simulink model "sim_switch_vol_hover"  (R2020b)
settings: Solver=VariableStepAuto  StartTime=0.0  StopTime=T  MaxStep=MaxStep  RelTol=RelTol
values from neighbouring files (symbols this model uses):
  a = 400    [switch_vol_hovering.m]
  b = 500    [switch_vol_hovering.m]
  drone = generateDarko()    [switch_vol_hovering.m]
  J = 200    [switch_vol_hovering.m]
  K_complet = [K(:,1:6), [0;0;0;0], K(:,7:12)]    [switch_vol_hovering.m]
  K_lin_control = [zeros(4,2), K_lin(:,1:4), zeros(4,1), K_lin(:,5:10)]    [switch_vol_hovering.m]
  position_cible = [50; 0; 0]    [switch_vol_hovering.m]
  rule = 1    [switch_vol_hovering.m]
  S_complet = [S(1:6,1:6), zeros(6,1), S(1:6,7:12); zeros(1,13); S(7:12,1:6), zeros(6,1), S(7:12,7:12)]    [switch_vol_hovering.m]
  T = 80    [switch_vol_hovering.m]
  u_eq_hover = drone.G*drone.MASS/(2*drone.Fb(1,1)) * [1;1;0;0]    [switch_vol_hovering.m]
  u_eq_vol = [trim(1);trim(1);trim(2);trim(2)]    [switch_vol_hovering.m]
  x0 = [p_initial; v_initial; q_initial; omega_initial; s]    [switch_vol_hovering.m]
  x_eq_hover = [[0; 0; 0]; [0; 0; 0]; [1/sqrt(2); 0; -1/sqrt(2);0]; [0; 0; 0]]    [switch_vol_hovering.m]
  x_eq_vol = [p_initial; v_initial; q_initial; omega_initial]    [switch_vol_hovering.m]
libraries: simulink x3, simulink_extras x3, aerolibanim x1, sharedtransform x1
settings Model: Creator=florian  LastModifiedBy=florian

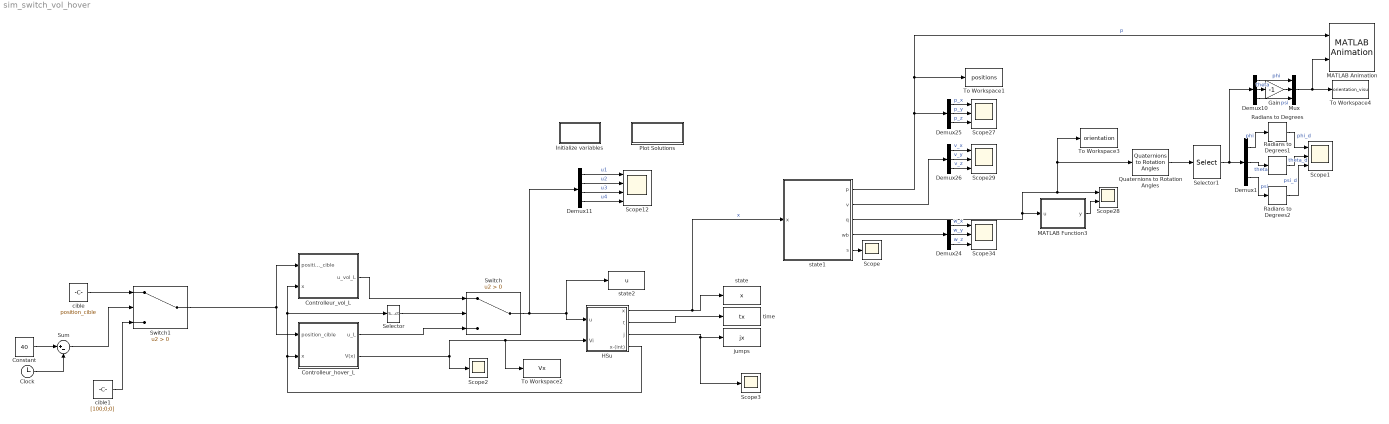
== system sim_switch_vol_hover ==
  Clock : Clock
  Constant : Constant  Value=40
  Controlleur_hover_L : Subsystem
  Controlleur_vol_L : Subsystem
  Demux{1,10,24..26} (5 alike) : Demux  Outputs=3
  Demux11 : Demux
  Gain : Gain  Gain=-1
  HSu : Subsystem  LoadFcn=set_param(gcb,'LinkStatus','none')
      settings: CopyFcn=|
      | set_param(gcb,'LinkStatus','none'),
      | set_param(gcs, 'MaxStep', 'MaxStep', 'RelTol', 'RelTol','Stop time', 'T')
      mask Display:
      | image(imread('Hcal.jpg'))
      | %plot([5 20 20 5 5],[5 5 20 20 5])
      | %text(8,13,'HyEq_mdl')
      | port_label('output', 1, 'x')
      | port_label('output', 2, 't')
      | port_label('output', 3, 'j')
      | port_label('output', 4, 'x-(int)')
      | port_label('input', 1, 'u')
      | port_label('input', 2, 'V(x)')
  Initialize variables : Subsystem  Priority=-10
      settings: OpenFcn=initialization_di
      mask Display: disp('Double Click\n to Initialize')
  MATLAB Animation : aerolibanim/MATLAB Animation  Tag=Matlab Animation 6 DOF  Vehicles=1  Geometries='astredwedge.mat'  BoundingBoxCoordinates=[-50,50,-50,50,-50,50]  CameraOffset=[-150,-50,0]  CameraViewAngle=3  SampleTime=0.2  FigurePosition=[962,411,639,384]
      settings: SourceProductBaseCode=AE
  MATLAB Function3 : MATLAB Function  TreatAsAtomicUnit=on
  Mux : Mux  Inputs=3
  Plot Solutions : Subsystem
      settings: OpenFcn=postprocessing_di
      mask Display: disp('Double Click to\n Plot Solutions')
  Quaternions to Rotation Angles : sharedtransform/Quaternions to Rotation Angles  rotationOrder=ZXY  aMode=aMode
      settings: SourceProductBaseCode=AE,PW,MT,UV,VE,VP
  Radians to Degrees : simulink_extras/Transformations/Radians to Degrees
  Radians to Degrees1 : simulink_extras/Transformations/Radians to Degrees
  Radians to Degrees2 : simulink_extras/Transformations/Radians to Degrees
  Scope : Scope
  Scope{1,27,29,34} (4 alike) : Scope  NumInputPorts=3
  Scope12 : Scope  NumInputPorts=4
  Scope2 : Scope
  Scope28 : Scope  NumInputPorts=2
  Scope3 : Scope
  Selector : Selector  InputPortWidth=14  IndexOptions=Index vector (dialog)  Indices=[14]  OutputSizes=1
  Selector1 : Selector  InputPortWidth=3  IndexOptions=Index vector (dialog)  Indices=[2 3 1]  OutputSizes=1
  Sum : Sum  Inputs=|+-
  Switch : Switch  Criteria=u2 > Threshold
  Switch1 : Switch  Criteria=u2 > Threshold
  To Workspace1 : ToWorkspace  VariableName=positions  SampleTime=-1
  To Workspace2 : ToWorkspace  VariableName=Vx  SampleTime=-1
  To Workspace3 : ToWorkspace  VariableName=orientation  SampleTime=-1
  To Workspace4 : ToWorkspace  VariableName=orientation_visu  SampleTime=-1
  cible : Constant  Value=position_cible
  cible1 : Constant  Value=[100;0;0]
  jumps : ToWorkspace  VariableName=jx  SampleTime=-1
  state : ToWorkspace  VariableName=x  SampleTime=-1
  state1 : MATLAB Function  TreatAsAtomicUnit=on
  state2 : ToWorkspace  VariableName=u  SampleTime=-1
  time : ToWorkspace  VariableName=tx  SampleTime=-1
  wires:
  Switch/1 -> HSu/1(u), state2/1, Demux11/1
  HSu/1(x) -> state1/1(x), state/1  "x"
  HSu/2(t) -> time/1
  HSu/3(j) -> jumps/1, Scope3/1
  Demux11/2 -> Scope12/2  "u2"
  Controlleur_vol_L/1(u_vol_L) -> Switch/1
  Controlleur_hover_L/1(u_L) -> Switch/3
  Demux11/1 -> Scope12/1  "u1"
  Demux11/4 -> Scope12/4  "u4"
  Switch1/1 -> Controlleur_vol_L/1(position_cible), Controlleur_hover_L/1(position_cible)
  Demux11/3 -> Scope12/3  "u3"
  Selector/1 -> Switch/2
  HSu/4(x-(int)) -> Controlleur_vol_L/2(x), Selector/1, Controlleur_hover_L/2(x)
  Demux1/2 -> Radians to Degrees1/1  "theta"
  Quaternions to Rotation Angles/1 -> Selector1/1
  Demux1/3 -> Radians to Degrees2/1  "psi"
  Demux24/2 -> Scope34/2  "w_y"
  Demux26/3 -> Scope29/3  "v_z"
  Demux25/3 -> Scope27/3  "p_z"
  Demux1/1 -> Radians to Degrees/1  "phi"
  Demux25/1 -> Scope27/1  "p_x"
  state1/3(q) -> Scope28/1, To Workspace3/1, Quaternions to Rotation Angles/1, MATLAB Function3/1(u)
  Radians to Degrees/1 -> Scope1/1  "phi_d"
  Radians to Degrees1/1 -> Scope1/2  "theta_d"
  Radians to Degrees2/1 -> Scope1/3  "psi_d"
  MATLAB Function3/1(y) -> Scope28/2
  state1/2(v) -> Demux26/1
  Demux26/2 -> Scope29/2  "v_y"
  Demux24/3 -> Scope34/3  "w_z"
  state1/4(wb) -> Demux24/1
  Demux24/1 -> Scope34/1  "w_x"
  Demux26/1 -> Scope29/1  "v_x"
  Demux25/2 -> Scope27/2  "p_y"
  state1/5(s) -> Scope/1
  cible/1 -> Switch1/1
  Constant/1 -> Sum/1
  Clock/1 -> Sum/2
  Sum/1 -> Switch1/2
  cible1/1 -> Switch1/3
  Controlleur_hover_L/2(V(x)) -> Scope2/1, To Workspace2/1, HSu/2(Vi)
  Gain/1 -> Mux/2
  Demux10/1 -> Mux/1  "phi"
  Demux10/2 -> Gain/1  "theta"
  Demux10/3 -> Mux/3  "psi"
  state1/1(p) -> MATLAB Animation/1, To Workspace1/1, Demux25/1  "p"
  Selector1/1 -> Demux10/1, Demux1/1
  Mux/1 -> To Workspace4/1, MATLAB Animation/2

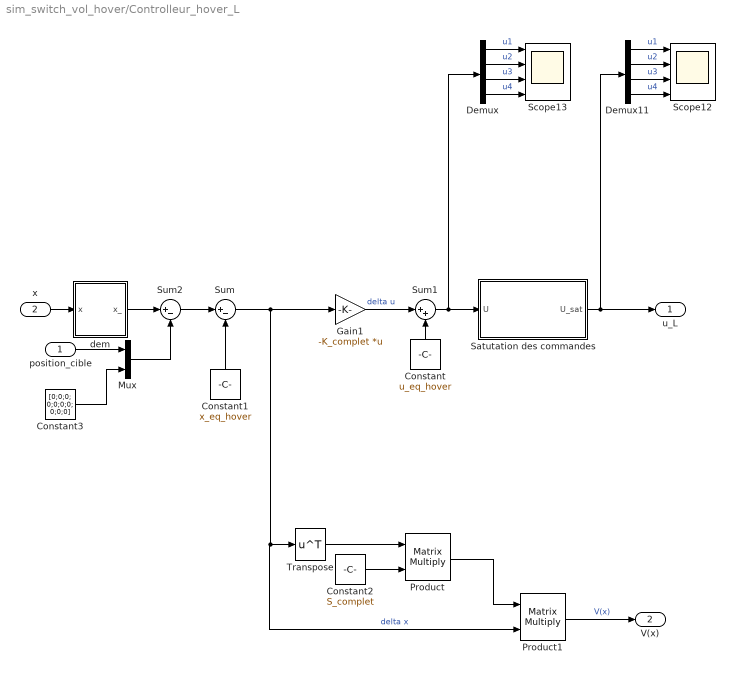
== system sim_switch_vol_hover/Controlleur_hover_L ==
  position_cible : Inport
  x : Inport  Port=2
  Constant : Constant  Value=u_eq_hover
  Constant1 : Constant  Value=x_eq_hover
  Constant2 : Constant  Value=S_complet
  Constant3 : Constant  Value=[0;0;0; 0;0;0;0; 0;0;0]
  Demux : Demux
  Demux11 : Demux
  Gain1 : Gain  Gain=-K_complet  Multiplication=Matrix(K*u) (u vector)
  Mux : Mux  Inputs=2
  Product : Product  Multiplication=Matrix(*)
  Product1 : Product  Multiplication=Matrix(*)
  Satutation des commandes : Subsystem
  Scope12 : Scope  NumInputPorts=4
  Scope13 : Scope  NumInputPorts=4
  Sum : Sum  Inputs=|+-
  Sum1 : Sum  Inputs=|++
  Sum2 : Sum  Inputs=|+-
  Transpose : Math  Operator=transpose  SaturateOnIntegerOverflow=on
  dem : MATLAB Function  TreatAsAtomicUnit=on
  u_L : Outport
  V(x) : Outport  Port=2
  wires:
  Demux/1 -> Scope13/1  "u1"
  Demux/3 -> Scope13/3  "u3"
  Gain1/1 -> Sum1/1  "delta u"
  Sum1/1 -> Satutation des commandes/1(U), Demux/1
  Sum/1 -> Gain1/1, Product1/2, Transpose/1  "delta x"
  Demux11/3 -> Scope12/3  "u3"
  Satutation des commandes/1(U_sat) -> u_L/1, Demux11/1
  Demux11/2 -> Scope12/2  "u2"
  Product1/1 -> V(x)/1  "V(x)"
  Demux/4 -> Scope13/4  "u4"
  Constant1/1 -> Sum/2
  Transpose/1 -> Product/1
  Product/1 -> Product1/1
  Constant/1 -> Sum1/2
  Demux11/4 -> Scope12/4  "u4"
  Demux/2 -> Scope13/2  "u2"
  Constant2/1 -> Product/2
  Sum2/1 -> Sum/1
  Demux11/1 -> Scope12/1  "u1"
  Mux/1 -> Sum2/2
  position_cible/1 -> Mux/1
  Constant3/1 -> Mux/2
  x/1 -> dem/1(x)
  dem/1(x_) -> Sum2/1

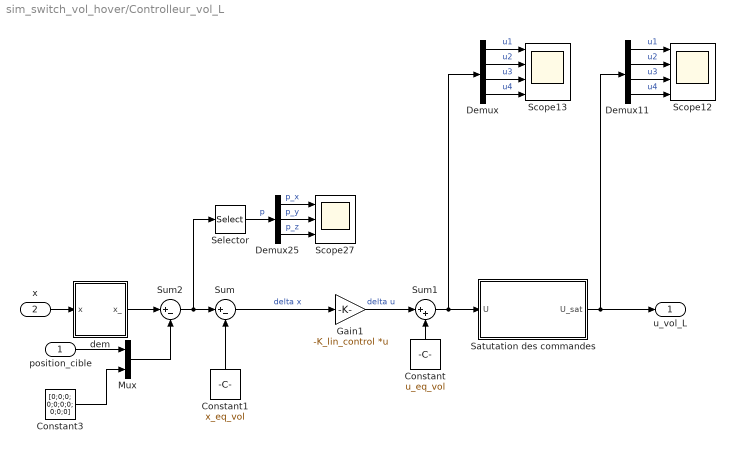
== system sim_switch_vol_hover/Controlleur_vol_L ==
  position_cible : Inport
  x : Inport  Port=2
  Constant : Constant  Value=u_eq_vol
  Constant1 : Constant  Value=x_eq_vol
  Constant3 : Constant  Value=[0;0;0; 0;0;0;0; 0;0;0]
  Demux : Demux
  Demux11 : Demux
  Demux25 : Demux  Outputs=3
  Gain1 : Gain  Gain=-K_lin_control  Multiplication=Matrix(K*u) (u vector)
  Mux : Mux  Inputs=2
  Satutation des commandes : Subsystem
  Scope12 : Scope  NumInputPorts=4
  Scope13 : Scope  NumInputPorts=4
  Scope27 : Scope  NumInputPorts=3
  Selector : Selector  InputPortWidth=13  IndexOptions=Index vector (dialog)  Indices=[1 2 3]  OutputSizes=1
  Sum : Sum  Inputs=|+-
  Sum1 : Sum  Inputs=|++
  Sum2 : Sum  Inputs=|+-
  dem : MATLAB Function  TreatAsAtomicUnit=on
  u_vol_L : Outport
  wires:
  Demux/1 -> Scope13/1  "u1"
  Demux/3 -> Scope13/3  "u3"
  Gain1/1 -> Sum1/1  "delta u"
  Sum1/1 -> Satutation des commandes/1(U), Demux/1
  Sum/1 -> Gain1/1  "delta x"
  Demux11/3 -> Scope12/3  "u3"
  Satutation des commandes/1(U_sat) -> u_vol_L/1, Demux11/1
  Demux11/2 -> Scope12/2  "u2"
  Demux/4 -> Scope13/4  "u4"
  Constant1/1 -> Sum/2
  Constant/1 -> Sum1/2
  Demux11/4 -> Scope12/4  "u4"
  Demux/2 -> Scope13/2  "u2"
  Sum2/1 -> Selector/1, Sum/1
  Demux11/1 -> Scope12/1  "u1"
  Mux/1 -> Sum2/2
  position_cible/1 -> Mux/1
  Constant3/1 -> Mux/2
  x/1 -> dem/1(x)
  dem/1(x_) -> Sum2/1
  Demux25/3 -> Scope27/3  "p_z"
  Demux25/1 -> Scope27/1  "p_x"
  Selector/1 -> Demux25/1  "p"
  Demux25/2 -> Scope27/2  "p_y"

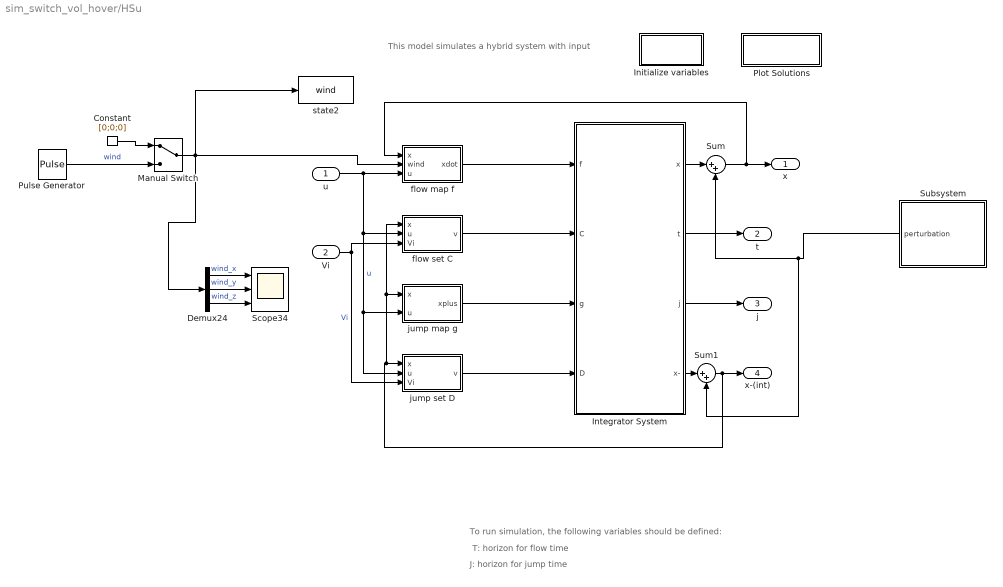
== system sim_switch_vol_hover/HSu ==
  note: J: horizon for jump time
  note: T: horizon for flow time
  note: To run simulation, the following variables should be defined:
  note: This model simulates a hybrid system with input
  u : Inport
  Vi : Inport  Port=2
  Constant : Constant  Value=[0;0;0]
  Demux24 : Demux  Outputs=3
  Initialize variables : Subsystem  Priority=-10
      settings: OpenFcn=|
      | try
      |      clearvars -except inifile pathfile_in pathfile_pos posfile
      |      cd(pathfile_in);
      |      eval(inifile);
      | catch
      |      [inifile,pathfile_in] = getInitializationfile;
      |      cd(pathfile_in);
      |      inifile = strrep(inifile,'.m','');
      |      eval(inifile);
      | end
      mask Display: disp('Double Click\n to Initialize')
  Integrator System : Subsystem  Priority=2  mask(Hybrid Integrator){T=T, J=J, x0=x0}
      mask prompts: T "Flow Horizon"; J "Jump Horizon"; x0 "Initial Condition"
      mask help:
      | This block integrates the state of the hybrid system defined by the flow map f (first input), the flow set C (second input), the jump map g (third input) and the jump set D (fourth input).
      | Starting from the initial condition x0 (last mask parameter), the system's state x evolves continuously within the set C, according to f(x,u), but is also subject to jumps within D, according to g(x,u).
      | The block also stops the simulation when the time t is greater than the flow horizon T (first mask parameter), or when the number of jumps j is greater than the jump horizon J (second mask parameter).
      | The outputs of the blocks are respectively x(t), t, j, x(t-).
      mask Help:
      | This block integrates the state of the hybrid system defined by the flow map f (first input), the flow set C (second input), the jump map g (third input) and the jump set D (fourth input).
      | <br>
      | Starting from the initial condition x0 (last mask parameter), the system's state x evolves continuously within the set C, according to f(x,u), but is also subject to jumps within D, according to g(x,u).
      | <br>
      | The block also stops the simulation when the time t is greater than the flow horizon T (first mask parameter), or when the number of jumps j is greater than the jump horizon J (second mask parameter).
      | <br>
      | The outputs of the blocks are respectively x(t), t, j, x(t-).
      | <br>
      | You can right click on the block and "Look under mask" to see what's inside the block.
      | Finally, refer to the manual (HybridSimulator_vXX.pdf) for more detailed information on how this hybrid simulator works.
  Manual Switch : ManualSwitch
  Plot Solutions : Subsystem
      settings: OpenFcn=|
      | try
      |      cd(pathfile_pos);
      |      eval(posfile);
      | catch
      |      [posfile,pathfile_pos] = getInitializationfile;
      |      cd(pathfile_pos);
      |      posfile = strrep(posfile,'.m','');
      |      eval(posfile);
      | end
      mask Display: disp('Double Click to\n Plot Solutions')
  Pulse Generator : DiscretePulseGenerator  PulseType=Time based  Amplitude=1.9  Period=10  PulseWidth=30  PhaseDelay=5
  Scope34 : Scope  NumInputPorts=3
  Subsystem : Subsystem
  Sum : Sum  Inputs=|++
  Sum1 : Sum  Inputs=|++
  flow map f : MATLAB Function  TreatAsAtomicUnit=on
  flow set C : MATLAB Function  TreatAsAtomicUnit=on
  jump map g : MATLAB Function  Priority=2  TreatAsAtomicUnit=on
  jump set D : MATLAB Function  TreatAsAtomicUnit=on
  state2 : ToWorkspace  VariableName=wind  SampleTime=-1
  x : Outport
  t : Outport  Port=2
  j : Outport  Port=3
  x-(int) : Outport  Port=4
  wires:
  jump map g/1(xplus) -> Integrator System/3(g)
  jump set D/1(v) -> Integrator System/4(D)
  u/1 -> jump set D/2(u), jump map g/2(u), flow set C/2(u), flow map f/3(u)  "u"
  Integrator System/3(j) -> j/1
  Integrator System/2(t) -> t/1
  flow set C/1(v) -> Integrator System/2(C)
  flow map f/1(xdot) -> Integrator System/1(f)
  Vi/1 -> jump set D/3(Vi), flow set C/3(Vi)  "Vi"
  Constant/1 -> Manual Switch/1
  Manual Switch/1 -> Demux24/1, state2/1, flow map f/2(wind)
  Demux24/1 -> Scope34/1  "wind_x"
  Demux24/2 -> Scope34/2  "wind_y"
  Demux24/3 -> Scope34/3  "wind_z"
  Pulse Generator/1 -> Manual Switch/2  "wind"
  Sum1/1 -> flow set C/1(x), jump map g/1(x), jump set D/1(x), x-(int)/1
  Subsystem/1(perturbation) -> Sum/2, Sum1/2
  Integrator System/1(x) -> Sum/1
  Sum/1 -> flow map f/1(x), x/1
  Integrator System/4(x-) -> Sum1/1

== system sim_switch_vol_hover/Initialize variables ==

== system sim_switch_vol_hover/Plot Solutions ==

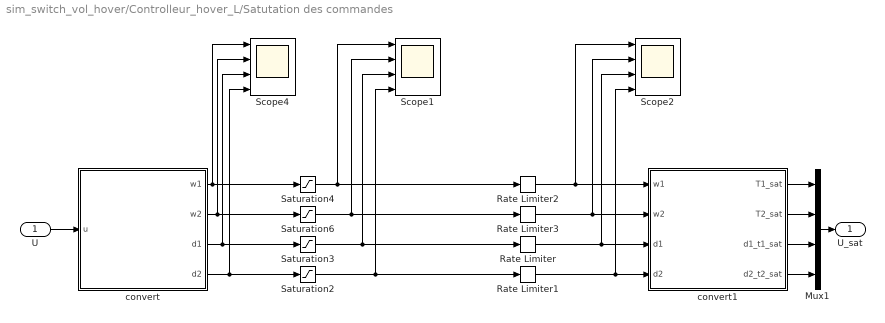
== system sim_switch_vol_hover/Controlleur_hover_L/Satutation des commandes ==
  U : Inport
  Mux1 : Mux
  Rate Limiter : RateLimiter  RisingSlewLimit=drone.ELEVON_RATE_CHANGE  FallingSlewLimit=-drone.ELEVON_RATE_CHANGE  SampleTimeMode=inherited
  Rate Limiter1 : RateLimiter  RisingSlewLimit=drone.ELEVON_RATE_CHANGE  FallingSlewLimit=-drone.ELEVON_RATE_CHANGE  SampleTimeMode=inherited
  Rate Limiter2 : RateLimiter  RisingSlewLimit=drone.MOTOR_RATE_CHANGE  FallingSlewLimit=-drone.MOTOR_RATE_CHANGE  SampleTimeMode=inherited
  Rate Limiter3 : RateLimiter  RisingSlewLimit=drone.MOTOR_RATE_CHANGE  FallingSlewLimit=-drone.MOTOR_RATE_CHANGE  SampleTimeMode=inherited
  Saturation2 : Saturate  UpperLimit=30*(pi/180)  LowerLimit=-30*(pi/180)
  Saturation3 : Saturate  UpperLimit=30*(pi/180)  LowerLimit=-30*(pi/180)
  Saturation4 : Saturate  UpperLimit=1000  LowerLimit=200
  Saturation6 : Saturate  UpperLimit=1000  LowerLimit=200
  Scope1 : Scope  NumInputPorts=4
  Scope2 : Scope  NumInputPorts=4
  Scope4 : Scope  NumInputPorts=4
  convert : MATLAB Function  TreatAsAtomicUnit=on
  convert1 : MATLAB Function  TreatAsAtomicUnit=on
  U_sat : Outport
  wires:
  convert/1(w1) -> Saturation4/1, Scope4/1
  Saturation3/1 -> Rate Limiter/1, Scope1/3
  convert/2(w2) -> Scope4/2, Saturation6/1
  convert/3(d1) -> Scope4/3, Saturation3/1
  convert/4(d2) -> Saturation2/1, Scope4/4
  convert1/1(T1_sat) -> Mux1/1
  convert1/4(d2_t2_sat) -> Mux1/4
  Mux1/1 -> U_sat/1
  convert1/2(T2_sat) -> Mux1/2
  convert1/3(d1_t1_sat) -> Mux1/3
  Saturation2/1 -> Rate Limiter1/1, Scope1/4
  Rate Limiter/1 -> Scope2/3, convert1/3(d1)
  Saturation6/1 -> Rate Limiter3/1, Scope1/2
  Saturation4/1 -> Rate Limiter2/1, Scope1/1
  Rate Limiter1/1 -> Scope2/4, convert1/4(d2)
  Rate Limiter2/1 -> Scope2/1, convert1/1(w1)
  Rate Limiter3/1 -> Scope2/2, convert1/2(w2)
  U/1 -> convert/1(u)

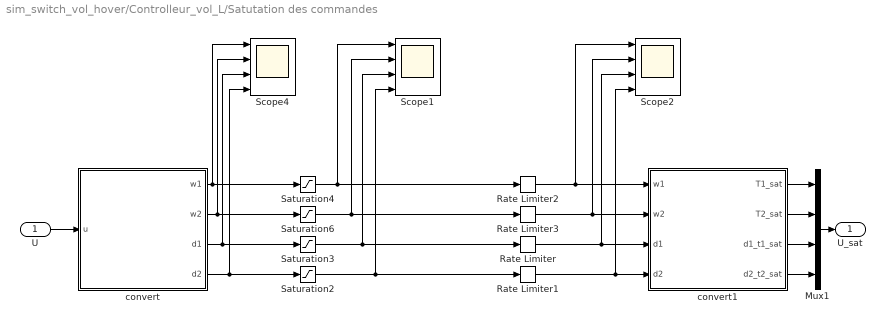
== system sim_switch_vol_hover/Controlleur_vol_L/Satutation des commandes ==
  U : Inport
  Mux1 : Mux
  Rate Limiter : RateLimiter  RisingSlewLimit=drone.ELEVON_RATE_CHANGE  FallingSlewLimit=-drone.ELEVON_RATE_CHANGE  SampleTimeMode=inherited
  Rate Limiter1 : RateLimiter  RisingSlewLimit=drone.ELEVON_RATE_CHANGE  FallingSlewLimit=-drone.ELEVON_RATE_CHANGE  SampleTimeMode=inherited
  Rate Limiter2 : RateLimiter  RisingSlewLimit=drone.MOTOR_RATE_CHANGE  FallingSlewLimit=-drone.MOTOR_RATE_CHANGE  SampleTimeMode=inherited
  Rate Limiter3 : RateLimiter  RisingSlewLimit=drone.MOTOR_RATE_CHANGE  FallingSlewLimit=-drone.MOTOR_RATE_CHANGE  SampleTimeMode=inherited
  Saturation2 : Saturate  UpperLimit=30*(pi/180)  LowerLimit=-30*(pi/180)
  Saturation3 : Saturate  UpperLimit=30*(pi/180)  LowerLimit=-30*(pi/180)
  Saturation4 : Saturate  UpperLimit=1000  LowerLimit=200
  Saturation6 : Saturate  UpperLimit=1000  LowerLimit=200
  Scope1 : Scope  NumInputPorts=4
  Scope2 : Scope  NumInputPorts=4
  Scope4 : Scope  NumInputPorts=4
  convert : MATLAB Function  TreatAsAtomicUnit=on
  convert1 : MATLAB Function  TreatAsAtomicUnit=on
  U_sat : Outport
  wires:
  convert/1(w1) -> Saturation4/1, Scope4/1
  Saturation3/1 -> Rate Limiter/1, Scope1/3
  convert/2(w2) -> Scope4/2, Saturation6/1
  convert/3(d1) -> Scope4/3, Saturation3/1
  convert/4(d2) -> Saturation2/1, Scope4/4
  convert1/1(T1_sat) -> Mux1/1
  convert1/4(d2_t2_sat) -> Mux1/4
  Mux1/1 -> U_sat/1
  convert1/2(T2_sat) -> Mux1/2
  convert1/3(d1_t1_sat) -> Mux1/3
  Saturation2/1 -> Rate Limiter1/1, Scope1/4
  Rate Limiter/1 -> Scope2/3, convert1/3(d1)
  Saturation6/1 -> Rate Limiter3/1, Scope1/2
  Saturation4/1 -> Rate Limiter2/1, Scope1/1
  Rate Limiter1/1 -> Scope2/4, convert1/4(d2)
  Rate Limiter2/1 -> Scope2/1, convert1/1(w1)
  Rate Limiter3/1 -> Scope2/2, convert1/2(w2)
  U/1 -> convert/1(u)

== system sim_switch_vol_hover/HSu/Initialize variables ==

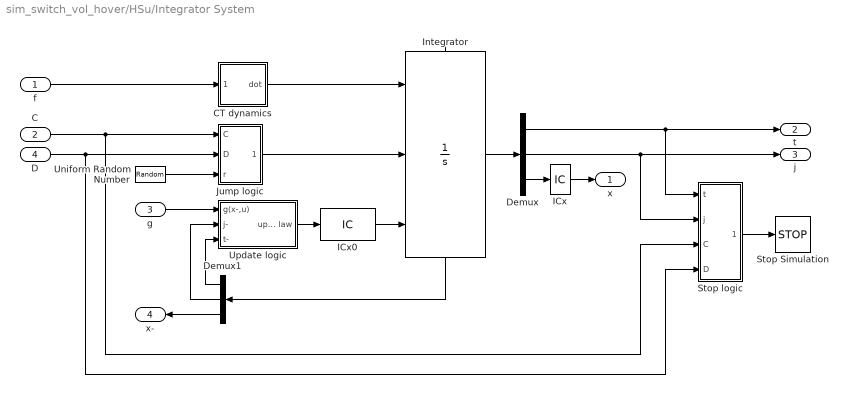
== system sim_switch_vol_hover/HSu/Integrator System ==
  f : Inport
  C : Inport  Port=2
  g : Inport  Port=3
  D : Inport  Port=4
  CT dynamics : Subsystem
  Demux : Demux  Outputs=[1 1 -1]
  Demux1 : Demux  Outputs=[1 1 -1]
  ICx : InitialCondition  Value=x0
  ICx0 : InitialCondition  Value=[0; 0; x0(:)]
  Integrator : Integrator  ExternalReset=level hold  InitialConditionSource=external  ShowStatePort=on  ZeroCross=off
  Jump logic : Subsystem
  Stop Simulation : Stop
  Stop logic : Subsystem
  Uniform Random Number : UniformRandomNumber  Minimum=0  Seed=abs(floor(100*rand))  SampleTime=0
  Update logic : Subsystem
  x : Outport
  t : Outport  Port=2
  j : Outport  Port=3
  x- : Outport  Port=4
  wires:
  ICx0/1 -> Integrator/3
  ICx/1 -> x/1
  Demux/3 -> ICx/1
  Integrator/State -> Demux1/1
  Demux/2 -> j/1, Stop logic/2(j)
  Demux/1 -> t/1, Stop logic/1(t)
  Update logic/1(update law) -> ICx0/1
  CT dynamics/1(dot) -> Integrator/1
  Stop logic/1(stop) -> Stop Simulation/1
  Integrator/1 -> Demux/1
  C/1 -> Stop logic/3(C), Jump logic/1(C)
  D/1 -> Stop logic/4(D), Jump logic/2(D)
  f/1 -> CT dynamics/1(f(x,u))
  Demux1/3 -> x-/1
  Jump logic/1(jump) -> Integrator/2
  Uniform Random Number/1 -> Jump logic/3(r)
  g/1 -> Update logic/1(g(x-,u))
  Demux1/1 -> Update logic/3(t-)
  Demux1/2 -> Update logic/2(j-)

== system sim_switch_vol_hover/HSu/Plot Solutions ==

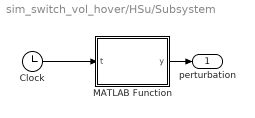
== system sim_switch_vol_hover/HSu/Subsystem ==
  Clock : Clock
  MATLAB Function : MATLAB Function  TreatAsAtomicUnit=on
  perturbation : Outport
  wires:
  Clock/1 -> MATLAB Function/1(t)
  MATLAB Function/1(y) -> perturbation/1

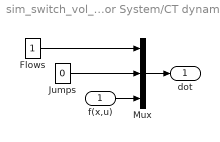
== system sim_switch_vol_hover/HSu/Integrator System/CT dynamics ==
  f(x,u) : Inport
  Flows : Constant
  Jumps : Constant  Value=0
  Mux : Mux  Inputs=[1 1 -1]
  dot : Outport
  wires:
  Jumps/1 -> Mux/2
  Flows/1 -> Mux/1
  Mux/1 -> dot/1
  f(x,u)/1 -> Mux/3

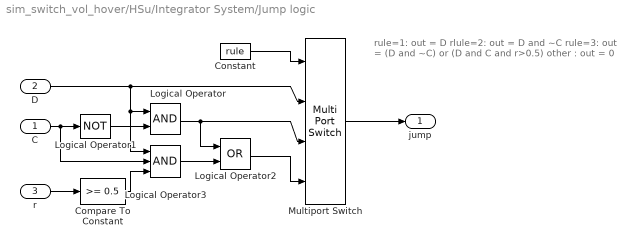
== system sim_switch_vol_hover/HSu/Integrator System/Jump logic ==
  note: rule=1:  out = D
      | rlule=2: out = D and ~C
      | rule=3:  out = (D and ~C)  or (D and C and r>0.5)
      | other :  out = 0
  C : Inport
  D : Inport  Port=2
  r : Inport  Port=3
  Compare To Constant : simulink/Logic and Bit Operations/Compare To Constant  relop=>=  const=0.5  OutDataTypeStr=uint8
  Constant : Constant  Value=rule
  Logical Operator : Logic  AllPortsSameDT=off  OutDataTypeStr=boolean
  Logical Operator1 : Logic  Operator=NOT  Inputs=1  AllPortsSameDT=off  OutDataTypeStr=boolean
  Logical Operator2 : Logic  Operator=OR  AllPortsSameDT=off  OutDataTypeStr=boolean
  Logical Operator3 : Logic  Inputs=3  AllPortsSameDT=off  OutDataTypeStr=boolean
  Multiport Switch : MultiPortSwitch
  jump : Outport
  wires:
  Constant/1 -> Multiport Switch/1
  D/1 -> Logical Operator3/1, Logical Operator/1, Multiport Switch/2
  r/1 -> Compare To Constant/1
  C/1 -> Logical Operator3/2, Logical Operator1/1
  Logical Operator1/1 -> Logical Operator/2
  Logical Operator/1 -> Multiport Switch/3, Logical Operator2/1
  Logical Operator2/1 -> Multiport Switch/4
  Multiport Switch/1 -> jump/1
  Compare To Constant/1 -> Logical Operator3/3
  Logical Operator3/1 -> Logical Operator2/2

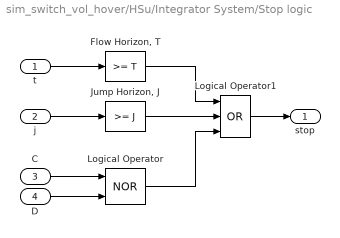
== system sim_switch_vol_hover/HSu/Integrator System/Stop logic ==
  t : Inport
  j : Inport  Port=2
  C : Inport  Port=3
  D : Inport  Port=4
  "Flow Horizon, T" : simulink/Logic and Bit Operations/Compare To Constant  relop=>=  const=T  OutDataTypeStr=uint8  ZeroCross=off
  "Jump Horizon, J" : simulink/Logic and Bit Operations/Compare To Constant  relop=>=  const=J  OutDataTypeStr=uint8  ZeroCross=off
  Logical Operator : Logic  Operator=NOR  AllPortsSameDT=off  OutDataTypeStr=boolean
  Logical Operator1 : Logic  Operator=OR  Inputs=3  AllPortsSameDT=off  OutDataTypeStr=boolean
  stop : Outport
  wires:
  "Flow Horizon, T"/1 -> Logical Operator1/1
  "Jump Horizon, J"/1 -> Logical Operator1/2
  Logical Operator/1 -> Logical Operator1/3
  D/1 -> Logical Operator/2
  t/1 -> "Flow Horizon, T"/1
  j/1 -> "Jump Horizon, J"/1
  C/1 -> Logical Operator/1
  Logical Operator1/1 -> stop/1

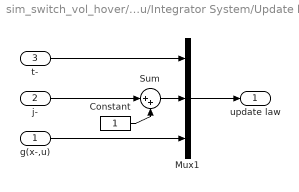
== system sim_switch_vol_hover/HSu/Integrator System/Update logic ==
  g(x-,u) : Inport
  j- : Inport  Port=2
  t- : Inport  Port=3
  Constant : Constant
  Mux1 : Mux  Inputs=[1 1 -1]
  Sum : Sum  Inputs=|++
  update law : Outport
  wires:
  Sum/1 -> Mux1/2
  Mux1/1 -> update law/1
  j-/1 -> Sum/1
  g(x-,u)/1 -> Mux1/3
  t-/1 -> Mux1/1
  Constant/1 -> Sum/2

== matlab function sim_switch_vol_hover/HSu/Subsystem/MATLAB Function ==
  data: t input; y output
function y = disturbance(t)
    if(t>10)

%         y = [50; zeros(13,1)];
        y = zeros(14,1);
    else
        y = zeros(14,1);
    end
end

== matlab function sim_switch_vol_hover/Controlleur_vol_L/Satutation des commandes/convert ==
  data: u input; w1 output; drone parameter; w2 output; d1 output; d2 output
function [w1, w2, d1, d2] = convert(u, drone)
%#codegen
kf = drone.PROP_KP;

T1 = max(u(1),0);
T2 = max(u(2),0);
d1_T1 = u(3);
d2_T2 = u(4);

w1 = sqrt(T1/kf);
w2 = sqrt(T2/kf);
d1 = d1_T1/T1;
d2 = d2_T2/T2;

== matlab function sim_switch_vol_hover/state1 ==
  data: x input; p output; v output; q output; wb output; s output
function [p, v,q, wb, s] = demux(x)
%#codegen

p = x(1:3);
v = x(4:6);
q  = x(7:10);
wb = x(11:13);
s = x(14);

== matlab function sim_switch_vol_hover/Controlleur_vol_L/Satutation des commandes/convert1 ==
  data: w1 input; w2 input; d1 input; d2 input; T1_sat output; T2_sat output; drone parameter; d1_t1_sat output; d2_t2_sat output
function [T1_sat, T2_sat, d1_t1_sat, d2_t2_sat] = convert2(w1, w2, d1, d2, drone)
%#codegen
kf = drone.PROP_KP;

T1_sat = kf*w1^2;
d1_t1_sat = d1*T1_sat;
T2_sat = kf*w2^2;
d2_t2_sat = d2*T2_sat;

== matlab function sim_switch_vol_hover/Controlleur_vol_L/dem ==
  data: x input; x_ output
function x_ = demux(x)

x_ = x(1:13);

== matlab function sim_switch_vol_hover/MATLAB Function3 ==
  data: u input; y output
function y = fcn(u)
%#codegen

y = norm(u);

== matlab function sim_switch_vol_hover/HSu/flow map f ==
  data: x input; wind input; xdot output; u input; drone parameter
function xdot = f(x, wind, u, drone)
%--------------------------------------------------------------------------
% Matlab M-file Project: HyEQ Toolbox @  Hybrid Systems Laboratory (HSL), 
% https://hybrid.soe.ucsc.edu/software
% http://hybridsimulator.wordpress.com/
%--------------------------------------------------------------------------
% Project: Simulation of a hybrid system
% Description: Flow map
%--------------------------------------------------------------------------
%--------------------------------------------------------------------------
%   See also HYEQSOLVER, PLOTARC, PLOTARC3, PLOTFLOWS, PLOTHARC,
%   PLOTHARCCOLOR, PLOTHARCCOLOR3D, PLOTHYBRIDARC, PLOTJUMPS.
%   Copyright @ Hybrid Systems Laboratory (HSL),
%   Revision: 0.0.0.3 Date: 05/20/2015 3:42:00
%--------------------------------------------------------------------------
% flow map: xdot=f(x,u);

%% physical constants
% gravity
g = drone.G;
% vehicle mass
m = drone.MASS;
% vehicle inertia matrix
J = drone.INERTIA; % [3x3 real symmetric] in body axis

%% state demultiplexing
% p = x(1:3);
v = x(4:6);
q  = x(7:10);
wb = x(11:13);
% s = x(14);

Rq = q2dcm(q);

[Fp, Mp] = external_force_moment(x, u, wind, drone);

% position
dpdt = v;

% kinematics
dvdt =  -[0;0;g] + (1/m)*Rq*drone.Fb*u + (1/m)*Rq*Fp; 

%% quaternion derivative
eta = q(1);
eps = q(2:4);

dqdt = (1/2)*[-eps'; eta*eye(3) + skew_sym(eps)]*wb;

%% angular velocity derivative
% kinematics
dwdt = -J\cross(wb, J*wb) + J\(drone.Mb*u) + J\Mp;


%% derivative multiplexing
xdot = [dpdt; dvdt; dqdt; dwdt; 0] ;

== matlab function sim_switch_vol_hover/HSu/flow set C ==
  data: x input; v output; u input; Vi input; a parameter; b parameter
function v   = C(x, u, Vi, a, b) 
%--------------------------------------------------------------------------
% Matlab M-file Project: HyEQ Toolbox @  Hybrid Systems Laboratory (HSL), 
% https://hybrid.soe.ucsc.edu/software
% http://hybridsimulator.wordpress.com/
%--------------------------------------------------------------------------
% Project: Simulation of a hybrid system
% Description: Flow set
%--------------------------------------------------------------------------
%--------------------------------------------------------------------------
%   See also HYEQSOLVER, PLOTARC, PLOTARC3, PLOTFLOWS, PLOTHARC,
%   PLOTHARCCOLOR, PLOTHARCCOLOR3D, PLOTHYBRIDARC, PLOTJUMPS.
%   Copyright @ Hybrid Systems Laboratory (HSL),
%   Revision: 0.0.0.3 Date: 05/20/2015 3:42:00
%
%state
s = x(14);


if (((Vi <= b ) && (s == 0)) || ((Vi >= a ) && (s == 1)))  % flow condition
    v = 1;  % report flow
else
    v = 0;   % do not report flow
end

== matlab function sim_switch_vol_hover/HSu/jump map g ==
  data: x input; xplus output; u input
function xplus = g(x, u)
%--------------------------------------------------------------------------
% Matlab M-file Project: HyEQ Toolbox @  Hybrid Systems Laboratory (HSL), 
% https://hybrid.soe.ucsc.edu/software
% http://hybridsimulator.wordpress.com/
%--------------------------------------------------------------------------
% Project: Simulation of a hybrid system
% Description: Jump map
%--------------------------------------------------------------------------
%--------------------------------------------------------------------------
%   See also HYEQSOLVER, PLOTARC, PLOTARC3, PLOTFLOWS, PLOTHARC,
%   PLOTHARCCOLOR, PLOTHARCCOLOR3D, PLOTHYBRIDARC, PLOTJUMPS.
%   Copyright @ Hybrid Systems Laboratory (HSL),
%   Revision: 0.0.0.3 Date: 05/20/2015 3:42:00
%--------------------------------------------------------------------------

xplus = [x(1:13); 1-x(14)];

== matlab function sim_switch_vol_hover/HSu/jump set D ==
  data: x input; v output; u input; Vi input; a parameter; b parameter
function v  = D(x, u, Vi, a, b) 
%--------------------------------------------------------------------------
% Matlab M-file Project: HyEQ Toolbox @  Hybrid Systems Laboratory (HSL), 
% https://hybrid.soe.ucsc.edu/software
% http://hybridsimulator.wordpress.com/
%--------------------------------------------------------------------------
% Project: Simulation of a hybrid system
% Description: Jump set
%--------------------------------------------------------------------------
%--------------------------------------------------------------------------
%   See also HYEQSOLVER, PLOTARC, PLOTARC3, PLOTFLOWS, PLOTHARC,
%   PLOTHARCCOLOR, PLOTHARCCOLOR3D, PLOTHYBRIDARC, PLOTJUMPS.
%   Copyright @ Hybrid Systems Laboratory (HSL),
%   Revision: 0.0.0.3 Date: 05/20/2015 3:42:00
%
%state
s = x(14);

if ( ((Vi >= b ) && (s == 0)) || ((Vi <= a ) && (s == 1)))  % jump condition
    v = 1;  % report jump
else
    v = 0;   % do not report jump
end

== matlab function sim_switch_vol_hover/Controlleur_hover_L/dem ==
  data: x input; x_ output
function x_ = demux(x)

x_ = x(1:13);

== matlab function sim_switch_vol_hover/Controlleur_hover_L/Satutation des commandes/convert ==
  data: u input; w1 output; drone parameter; w2 output; d1 output; d2 output
function [w1, w2, d1, d2] = convert(u, drone)
%#codegen
kf = drone.PROP_KP;

T1 = max(u(1),0);
T2 = max(u(2),0);
d1_T1 = u(3);
d2_T2 = u(4);

w1 = sqrt(T1/kf);
w2 = sqrt(T2/kf);
d1 = d1_T1/T1;
d2 = d2_T2/T2;

== matlab function sim_switch_vol_hover/Controlleur_hover_L/Satutation des commandes/convert1 ==
  data: w1 input; w2 input; d1 input; d2 input; T1_sat output; T2_sat output; drone parameter; d1_t1_sat output; d2_t2_sat output
function [T1_sat, T2_sat, d1_t1_sat, d2_t2_sat] = convert2(w1, w2, d1, d2, drone)
%#codegen
kf = drone.PROP_KP;

T1_sat = kf*w1^2;
d1_t1_sat = d1*T1_sat;
T2_sat = kf*w2^2;
d2_t2_sat = d2*T2_sat;
